simulink model "controlMCUSlugsMKII"  (Simulink 6.6)
settings: Solver=FixedStepDiscrete  StartTime=0.0  StopTime=10.0  FixedStep=0.01  RelTol=1e-3
InitFcn:
  | mcuInit
values from neighbouring files (symbols this model uses):
  apSampleTime = 0.01    [mcuInit.m]
  derivativesConstant = 5    [mcuInit.m]
  T = 0.01    [mcuInit.m]
undefined symbols (not defined in the file or in its folder): bankCommandLimit, baseHeight, bda, bde, bdr, bdt, bICda, bICde, bICdr, bICdt, controlMCUInit, daLimit, deLimit, drLimit, dtLimit, getAccBias, getAccels, getAttitude, getMidLevelCommands, getPassValues, getPidIdx, getVned, getWP, getXYZ, gsRead, ISA_g, lowRateTelemetryMavlink, mda, mde, mdr, mdt, mICda, mICde, mICdr, mICdt, pitchCommandLimit, protDecodeMavlink, readIpc, send2GS, setCurrentCommands, setDiagnosticFloat, setDiagnosticShort, setLogFloat1, setLogFloat2, setNavLat, setNavLong, setNavNav, u1, u2, updateEuler, updateLoad, updatePQR, updatePWM, updatePWM2, y1
libraries: dsPICdrivers x85, simulink x79, SLUGS_Library x23, aerolibconvert2 x5, aerolibutil x3
(part 5 of 5)

== system controlMCUSlugsMKII/Inner Loop/ Navigation/Navigation/Park, Deyst & How Lat Accel Cmd/GainSchedule L2 and Get Groundspeed/Norm  ==
  Vector : Inport
  Square Vx and Vy  Only. Vz is not considered CAREFUL : Subsystem  AncestorBlock=SLUGS_Library/Subsystem3
  Subsystem1 : SLUGS_Library/Subsystem1  SystemSampleTime=-1
  "[-25 25]" : Saturate  UpperLimit=25  LowerLimit=-25  SampleTime=.01
  Norm : Outport
  wires:
  Subsystem1/1 -> Norm/1
  Vector/1 -> "[-25 25]"/1
  Square Vx and Vy  Only. Vz is not considered CAREFUL/1(x dot y) -> Subsystem1/1
  "[-25 25]"/1 -> Square Vx and Vy  Only. Vz is not considered CAREFUL/1(x), Square Vx and Vy  Only. Vz is not considered CAREFUL/2(y)

== system controlMCUSlugsMKII/Inner Loop/ Navigation/Navigation/Park, Deyst & How Lat Accel Cmd/GainSchedule L2 and Get Groundspeed/Protect NaNs ==
  In1 : Inport
  Integer Delay3 : simulink/Discrete/Integer Delay  Orientation=left  vinit=0.0  samptime=T  NumDelays=1
  Relational Operator2 : RelationalOperator  Operator===  LogicOutDataTypeMode=Specify via dialog
  Switch3 : Switch  Criteria=u2 > Threshold  Threshold=0.3  SampleTime=.01
  Out1 : Outport  Orientation=down
  wires:
  Relational Operator2/1 -> Switch3/2
  In1/1 -> Switch3/1, Relational Operator2/1, Relational Operator2/2
  Switch3/1 -> Integer Delay3/1, Out1/1
  Integer Delay3/1 -> Switch3/3

== system controlMCUSlugsMKII/Inner Loop/ Navigation/Navigation/Park, Deyst & How Lat Accel Cmd/Park's Lateral Accel Command/Protect NaNs ==
  In1 : Inport
  Integer Delay3 : simulink/Discrete/Integer Delay  Orientation=left  vinit=0.0  samptime=T  NumDelays=1
  Relational Operator2 : RelationalOperator  Operator===  LogicOutDataTypeMode=Specify via dialog
  Switch3 : Switch  Criteria=u2 > Threshold  Threshold=0.3  SampleTime=.01
  Out1 : Outport  Orientation=down
  wires:
  Relational Operator2/1 -> Switch3/2
  In1/1 -> Switch3/1, Relational Operator2/1, Relational Operator2/2
  Switch3/1 -> Integer Delay3/1, Out1/1
  Integer Delay3/1 -> Switch3/3

== system controlMCUSlugsMKII/Inner Loop/ Navigation/Navigation/Compute WP Index/Compute P/Compute T  in Frenet/Normalize Vector ==
  Vector : Inport
  Divide : Product  Inputs=*/  OutScaling=2^-10
  Norm : Subsystem  AncestorBlock=SLUGS_Library/Navigation/Norm
  Zero Bound : Saturate  UpperLimit=inf  LowerLimit=0.001
  Normalized : Outport
  wires:
  Divide/1 -> Normalized/1
  Zero Bound/1 -> Divide/2
  Norm/1(Norm) -> Zero Bound/1
  Vector/1 -> Divide/1, Norm/1(Vector)

== system controlMCUSlugsMKII/Inner Loop/ Navigation/Navigation/Compute WP Index/Compute P/Geod2LTP1/ECEF2LTP (UEN) ==
  ECEF coordinates : Inport
  "Long, Lat" : Inport  Port=2
  Deg2R : Gain  Gain=pi/180  SaturateOnIntegerOverflow=on
  Demux3 : Demux  Outputs=2
  From Body to Universal1 : Subsystem
  Product1 : Product  Multiplication=Matrix(*)  SaturateOnIntegerOverflow=on  InputSameDT=on
  Out : Outport
  wires:
  "Long, Lat"/1 -> Deg2R/1
  Product1/1 -> Out/1
  Demux3/2 -> From Body to Universal1/2(lat)
  Demux3/1 -> From Body to Universal1/1(long)
  Deg2R/1 -> Demux3/1
  ECEF coordinates/1 -> Product1/2
  From Body to Universal1/1(DCM) -> Product1/1

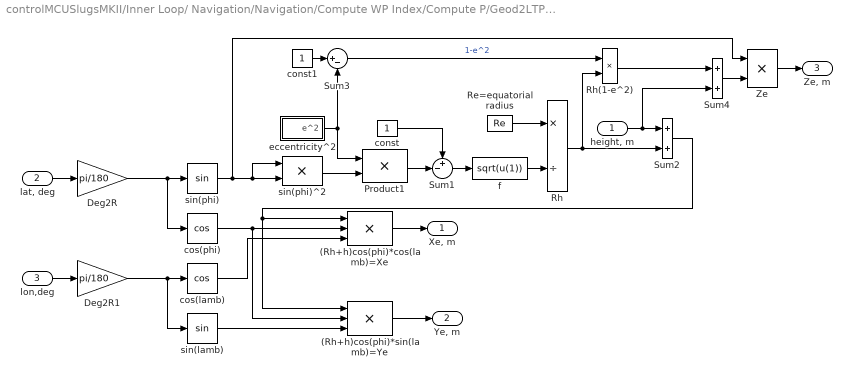
== system controlMCUSlugsMKII/Inner Loop/ Navigation/Navigation/Compute WP Index/Compute P/Geod2LTP1/Geod2ECEF1 ==
  "height, m" : Inport
  "lat, deg" : Inport  Port=2
  lon,deg : Inport  Port=3
  (Rh+h)cos(phi)*cos(lamb)=Xe : Product  Inputs=3  OutDataTypeMode=single  SaturateOnIntegerOverflow=on  InputSameDT=on
  (Rh+h)cos(phi)*sin(lamb)=Ye : Product  Inputs=3  OutDataTypeMode=single  SaturateOnIntegerOverflow=on  InputSameDT=on
  Deg2R : Gain  Gain=pi/180  OutDataTypeMode=Specify via dialog  OutDataType=float('single')  SaturateOnIntegerOverflow=on
  Deg2R1 : Gain  Gain=pi/180  OutDataTypeMode=Specify via dialog  OutDataType=float('single')  SaturateOnIntegerOverflow=on
  Product1 : Product  SaturateOnIntegerOverflow=on  InputSameDT=on
  Re=equatorial radius : Constant  Value=Re  OutDataTypeMode=single
  Rh : Product  Inputs=*/  OutDataTypeMode=single  SaturateOnIntegerOverflow=on  InputSameDT=on
  Rh(1-e^2) : Product  OutDataTypeMode=single  SaturateOnIntegerOverflow=on  InputSameDT=on
  Sum1 : Sum  Inputs=+-|  SaturateOnIntegerOverflow=on  InputSameDT=on
  Sum2 : Sum  SaturateOnIntegerOverflow=on  InputSameDT=on
      settings: AttributesFormatString=Rh+h
  Sum3 : Sum  Inputs=|+-  SaturateOnIntegerOverflow=on  InputSameDT=on
  Sum4 : Sum  OutDataTypeMode=single  SaturateOnIntegerOverflow=on  InputSameDT=on
      settings: AttributesFormatString=(1-e^2)Rh+h
  Ze : Product  OutDataTypeMode=single  SaturateOnIntegerOverflow=on  InputSameDT=on
  const : Constant  OutDataTypeMode=single
  const1 : Constant  OutDataTypeMode=single
  cos(lamb) : Trigonometry  Operator=cos
  cos(phi) : Trigonometry  Operator=cos
  eccentricity^2 : Subsystem
  f : Fcn  Expr=sqrt(u(1))
  sin(lamb) : Trigonometry
  sin(phi) : Trigonometry
  sin(phi)^2 : Product  SaturateOnIntegerOverflow=on  InputSameDT=on
  "Xe, m " : Outport
  "Ye, m " : Outport  Port=2
  "Ze, m " : Outport  Port=3
  wires:
  "lat, deg"/1 -> Deg2R/1
  sin(phi)/1 -> sin(phi)^2/1, sin(phi)^2/2, Ze/1
  f/1 -> Rh/2
  Re=equatorial radius/1 -> Rh/1
  Rh/1 -> Sum2/2, Rh(1-e^2)/2
  Product1/1 -> Sum1/2
  Sum1/1 -> f/1
  const/1 -> Sum1/1
  "height, m"/1 -> Sum4/2, Sum2/1
  eccentricity^2/1(e^2) -> Product1/1, Sum3/2
  sin(phi)^2/1 -> Product1/2
  const1/1 -> Sum3/1
  Sum3/1 -> Rh(1-e^2)/1  "1-e^2"
  Rh(1-e^2)/1 -> Sum4/1
  Sum4/1 -> Ze/2
  lon,deg/1 -> Deg2R1/1
  cos(phi)/1 -> (Rh+h)cos(phi)*cos(lamb)=Xe/2, (Rh+h)cos(phi)*sin(lamb)=Ye/2
  cos(lamb)/1 -> (Rh+h)cos(phi)*cos(lamb)=Xe/3
  sin(lamb)/1 -> (Rh+h)cos(phi)*sin(lamb)=Ye/3
  Ze/1 -> "Ze, m "/1
  Deg2R/1 -> cos(phi)/1, sin(phi)/1
  Deg2R1/1 -> cos(lamb)/1, sin(lamb)/1
  Sum2/1 -> (Rh+h)cos(phi)*sin(lamb)=Ye/1, (Rh+h)cos(phi)*cos(lamb)=Xe/1
  (Rh+h)cos(phi)*cos(lamb)=Xe/1 -> "Xe, m "/1
  (Rh+h)cos(phi)*sin(lamb)=Ye/1 -> "Ye, m "/1

== system controlMCUSlugsMKII/Inner Loop/ Navigation/Navigation/Compute WP Index/Compute P/Get Circles/Compute CCW Angle From 2 Vectors ==
  U : Inport
  V : Inport  Port=2
  Add : Sum  Inputs=+-  OutScaling=2^-10
  Embedded MATLAB Function1 : Stateflow chart
  Selector : Selector  IndexOptions=Index vector (dialog)  Indices=[1]  OutputSizes=1  InputPortWidth=3
  Selector1 : Selector  IndexOptions=Index vector (dialog)  Indices=[1]  OutputSizes=1  InputPortWidth=3
  Selector2 : Selector  IndexOptions=Index vector (dialog)  Indices=[2]  OutputSizes=1  InputPortWidth=3
  Selector3 : Selector  IndexOptions=Index vector (dialog)  Indices=[2]  OutputSizes=1  InputPortWidth=3
  Subsystem1 : SLUGS_Library/Subsystem4  SystemSampleTime=-1
  Subsystem4 : SLUGS_Library/Subsystem4  SystemSampleTime=-1
  CCW Ang : Outport
  wires:
  Embedded MATLAB Function1/1(angle) -> CCW Ang/1
  V/1 -> Selector1/1, Selector2/1
  U/1 -> Selector/1, Selector3/1
  Add/1 -> Embedded MATLAB Function1/1(rawAngle)
  Subsystem1/1 -> Add/2
  Subsystem4/1 -> Add/1
  Selector1/1 -> Subsystem1/2
  Selector2/1 -> Subsystem1/1
  Selector/1 -> Subsystem4/2
  Selector3/1 -> Subsystem4/1

== system controlMCUSlugsMKII/Inner Loop/ Navigation/Navigation/Compute WP Index/Compute P/Get Circles/Compute delta Left Turn ==
  gamma : Inport
  Enable : EnablePort
  Add : Sum  Inputs=+-  OutDataTypeMode=single  OutScaling=2^-10
  Constant1 : Constant  Value=2  OutDataTypeMode=single
  Constant5 : Constant  Value=pi  OutDataTypeMode=single
  Divide : Product  Inputs=*/  OutDataTypeMode=single  OutScaling=2^-10
  Gain : Gain  Gain=-1
  delta : Outport
  wires:
  Gain/1 -> delta/1
  Add/1 -> Divide/1
  gamma/1 -> Add/2
  Constant5/1 -> Add/1
  Divide/1 -> Gain/1
  Constant1/1 -> Divide/2

== system controlMCUSlugsMKII/Inner Loop/ Navigation/Navigation/Compute WP Index/Compute P/Get Circles/compute delta Right Turn ==
  gamma : Inport
  Enable : EnablePort
  Add : Sum  Inputs=-+  OutDataTypeMode=single  OutScaling=2^-10
  Constant1 : Constant  Value=2  OutDataTypeMode=single
  Constant5 : Constant  Value=pi  OutDataTypeMode=single
  Divide : Product  Inputs=*/  OutDataTypeMode=single  OutScaling=2^-10
  delta : Outport
  wires:
  Divide/1 -> delta/1  "delta"
  gamma/1 -> Add/2
  Constant1/1 -> Divide/2
  Add/1 -> Divide/1
  Constant5/1 -> Add/1

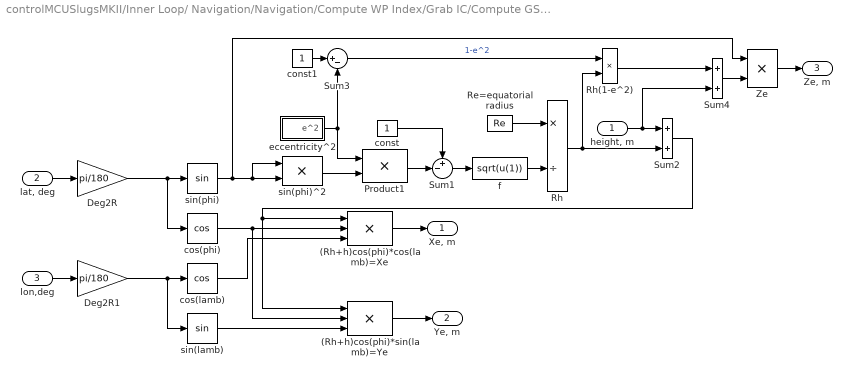
== system controlMCUSlugsMKII/Inner Loop/ Navigation/Navigation/Compute WP Index/Grab IC/Compute GS Location/Geod2ECEF1 ==
  "height, m" : Inport
  "lat, deg" : Inport  Port=2
  lon,deg : Inport  Port=3
  (Rh+h)cos(phi)*cos(lamb)=Xe : Product  Inputs=3  OutDataTypeMode=single  SaturateOnIntegerOverflow=on  InputSameDT=on
  (Rh+h)cos(phi)*sin(lamb)=Ye : Product  Inputs=3  OutDataTypeMode=single  SaturateOnIntegerOverflow=on  InputSameDT=on
  Deg2R : Gain  Gain=pi/180  OutDataTypeMode=Specify via dialog  OutDataType=float('single')  SaturateOnIntegerOverflow=on
  Deg2R1 : Gain  Gain=pi/180  OutDataTypeMode=Specify via dialog  OutDataType=float('single')  SaturateOnIntegerOverflow=on
  Product1 : Product  SaturateOnIntegerOverflow=on  InputSameDT=on
  Re=equatorial radius : Constant  Value=Re  OutDataTypeMode=single
  Rh : Product  Inputs=*/  OutDataTypeMode=single  SaturateOnIntegerOverflow=on  InputSameDT=on
  Rh(1-e^2) : Product  OutDataTypeMode=single  SaturateOnIntegerOverflow=on  InputSameDT=on
  Sum1 : Sum  Inputs=+-|  SaturateOnIntegerOverflow=on  InputSameDT=on
  Sum2 : Sum  SaturateOnIntegerOverflow=on  InputSameDT=on
      settings: AttributesFormatString=Rh+h
  Sum3 : Sum  Inputs=|+-  SaturateOnIntegerOverflow=on  InputSameDT=on
  Sum4 : Sum  OutDataTypeMode=single  SaturateOnIntegerOverflow=on  InputSameDT=on
      settings: AttributesFormatString=(1-e^2)Rh+h
  Ze : Product  OutDataTypeMode=single  SaturateOnIntegerOverflow=on  InputSameDT=on
  const : Constant  OutDataTypeMode=single
  const1 : Constant  OutDataTypeMode=single
  cos(lamb) : Trigonometry  Operator=cos
  cos(phi) : Trigonometry  Operator=cos
  eccentricity^2 : Subsystem
  f : Fcn  Expr=sqrt(u(1))
  sin(lamb) : Trigonometry
  sin(phi) : Trigonometry
  sin(phi)^2 : Product  SaturateOnIntegerOverflow=on  InputSameDT=on
  "Xe, m " : Outport
  "Ye, m " : Outport  Port=2
  "Ze, m " : Outport  Port=3
  wires:
  "lat, deg"/1 -> Deg2R/1
  sin(phi)/1 -> sin(phi)^2/1, sin(phi)^2/2, Ze/1
  f/1 -> Rh/2
  Re=equatorial radius/1 -> Rh/1
  Rh/1 -> Sum2/2, Rh(1-e^2)/2
  Product1/1 -> Sum1/2
  Sum1/1 -> f/1
  const/1 -> Sum1/1
  "height, m"/1 -> Sum4/2, Sum2/1
  eccentricity^2/1(e^2) -> Product1/1, Sum3/2
  sin(phi)^2/1 -> Product1/2
  const1/1 -> Sum3/1
  Sum3/1 -> Rh(1-e^2)/1  "1-e^2"
  Rh(1-e^2)/1 -> Sum4/1
  Sum4/1 -> Ze/2
  lon,deg/1 -> Deg2R1/1
  cos(phi)/1 -> (Rh+h)cos(phi)*cos(lamb)=Xe/2, (Rh+h)cos(phi)*sin(lamb)=Ye/2
  cos(lamb)/1 -> (Rh+h)cos(phi)*cos(lamb)=Xe/3
  sin(lamb)/1 -> (Rh+h)cos(phi)*sin(lamb)=Ye/3
  Ze/1 -> "Ze, m "/1
  Deg2R/1 -> cos(phi)/1, sin(phi)/1
  Deg2R1/1 -> cos(lamb)/1, sin(lamb)/1
  Sum2/1 -> (Rh+h)cos(phi)*sin(lamb)=Ye/1, (Rh+h)cos(phi)*cos(lamb)=Xe/1
  (Rh+h)cos(phi)*cos(lamb)=Xe/1 -> "Xe, m "/1
  (Rh+h)cos(phi)*sin(lamb)=Ye/1 -> "Ye, m "/1

== system controlMCUSlugsMKII/Inner Loop/ Navigation/Navigation/Compute WP Index/Switch when  in Line Segment/Compute  Projection/Protect NaNs ==
  In1 : Inport
  Integer Delay3 : simulink/Discrete/Integer Delay  Orientation=left  vinit=0.0  samptime=T  NumDelays=1
  Relational Operator2 : RelationalOperator  Operator===  LogicOutDataTypeMode=Specify via dialog
  Switch3 : Switch  Criteria=u2 > Threshold  Threshold=0.3  SampleTime=.01
  Out1 : Outport  Orientation=down
  wires:
  Relational Operator2/1 -> Switch3/2
  In1/1 -> Switch3/1, Relational Operator2/1, Relational Operator2/2
  Switch3/1 -> Integer Delay3/1, Out1/1
  Integer Delay3/1 -> Switch3/3

== system controlMCUSlugsMKII/Inner Loop/ Navigation/Navigation/Compute WP Index/Switch when  in Line Segment/Compute  Projection/Subsystem3 ==
  x : Inport
  y : Inport  Port=2
  Embedded MATLAB Function : Stateflow chart
  x dot y : Outport
  wires:
  Embedded MATLAB Function/1(xDoty) -> x dot y/1
  x/1 -> Embedded MATLAB Function/1(x)
  y/1 -> Embedded MATLAB Function/2(y)

== system controlMCUSlugsMKII/Inner Loop/ Navigation/Navigation/Compute WP Index/Switch when  in Line Segment/Compute Total Run/Compute Distance ==
  Pos 1 : Inport
  Pos 2 : Inport  Port=2
  Add : Sum  Inputs=+-  OutScaling=2^-10
  Norm : Subsystem  AncestorBlock=SLUGS_Library/Navigation/Norm
  Dist : Outport
  wires:
  Norm/1(Norm) -> Dist/1
  Add/1 -> Norm/1(Vector)
  Pos 2/1 -> Add/2
  Pos 1/1 -> Add/1

== system controlMCUSlugsMKII/Inner Loop/ Navigation/Navigation/Compute WP Index/Switch when  in Line Segment/Compute Total Run/Protect NaNs ==
  In1 : Inport
  Integer Delay3 : simulink/Discrete/Integer Delay  Orientation=left  vinit=0.0  samptime=T  NumDelays=1
  Relational Operator2 : RelationalOperator  Operator===  LogicOutDataTypeMode=Specify via dialog
  Switch3 : Switch  Criteria=u2 > Threshold  Threshold=0.3  SampleTime=.01
  Out1 : Outport  Orientation=down
  wires:
  Relational Operator2/1 -> Switch3/2
  In1/1 -> Switch3/1, Relational Operator2/1, Relational Operator2/2
  Switch3/1 -> Integer Delay3/1, Out1/1
  Integer Delay3/1 -> Switch3/3

== system controlMCUSlugsMKII/Inner Loop/ Navigation/Navigation/Compute WP Index/Switch when  in Line Segment/WP Update/Detect Change ==
  Data : Inport
  Difference1 : simulink/Discrete/Difference  SystemSampleTime=-1  ICPrevInput=0.0  OutDataType=sfix(16)  OutScaling=2^-10  DoSatur=off
  Saturation1 : Saturate  UpperLimit=1  LowerLimit=0  SampleTime=T
  Subsystem9 : SLUGS_Library/Subsystem9  SystemSampleTime=-1
  change? : Outport
  wires:
  Subsystem9/1 -> Saturation1/1
  Saturation1/1 -> change?/1
  Data/1 -> Difference1/1
  Difference1/1 -> Subsystem9/1

== system controlMCUSlugsMKII/Inner Loop/ Navigation/Navigation/Compute WP Index/Switch when  in Line Segment/WP Update/Detect Change1 ==
  Data : Inport
  Difference1 : simulink/Discrete/Difference  SystemSampleTime=-1  ICPrevInput=0.0  OutDataType=sfix(16)  OutScaling=2^-10  DoSatur=off
  Saturation1 : Saturate  UpperLimit=1  LowerLimit=0  SampleTime=T
  Subsystem9 : SLUGS_Library/Subsystem9  SystemSampleTime=-1
  change? : Outport
  wires:
  Difference1/1 -> Subsystem9/1
  Data/1 -> Difference1/1
  Saturation1/1 -> change?/1
  Subsystem9/1 -> Saturation1/1

== system controlMCUSlugsMKII/Inner Loop/ Navigation/Navigation/Compute WP Index/Switch when  in Line Segment/WP Update/Detect Change2 ==
  Data : Inport
  Difference1 : simulink/Discrete/Difference  SystemSampleTime=-1  ICPrevInput=0.0  OutDataType=sfix(16)  OutScaling=2^-10  DoSatur=off
  Saturation1 : Saturate  UpperLimit=1  LowerLimit=0  SampleTime=T
  Subsystem9 : SLUGS_Library/Subsystem9  SystemSampleTime=-1
  change? : Outport
  wires:
  Subsystem9/1 -> Saturation1/1
  Saturation1/1 -> change?/1
  Data/1 -> Difference1/1
  Difference1/1 -> Subsystem9/1

== system controlMCUSlugsMKII/Inner Loop/ Navigation/Navigation/Get Wps Compute Frenet/Geod2LTP1/ECEF2LTP (UEN)/From Body to Universal1 ==
  long : Inport
  lat : Inport  Port=2
  Mux : Mux  Inputs=2
  Reshape 9x1->3x1 : S-Function  FunctionName=sreshape  Parameters=OutputDimensionality, OutputDimensions  mask(Reshape){OutputDimensionality=Customize, OutputDimensions=[3,3]}
      mask prompts: OutputDimensionality "Output dimensionality:"; OutputDimensions "Output dimensions:"
      mask help:
      | Change the dimensions of a vector or matrix input signal. Output
      |  - a one-dimensional array (vector),
      |  - a column vector (Mx1 matrix),
      |  - a row vector (1xN matrix), or
      |  - a matrix or vector with specified dimensions, e.g., [M, N] or [W].
      mask init:
      | s = reshapemask(gcb,'init');
      mask StyleString: popup(1-D array|Column vector|Row vector|Customize),edit
      mask CallbackString: reshapemask(gcb,'cbDimensionality')|
      mask Display: disp('Reshape')
  Rotation Matrix from Long//Lat : Subsystem
      mask Type: Vector Transformation
      mask Description: Vector Transformation
      mask Display: disp('axis')
  DCM : Outport
  wires:
  lat/1 -> Mux/2
  long/1 -> Mux/1
  Mux/1 -> Rotation Matrix from Long//Lat/1(long lat)
  Rotation Matrix from Long//Lat/1(DCM) -> Reshape 9x1->3x1/1
  Reshape 9x1->3x1/1 -> DCM/1

== system controlMCUSlugsMKII/Inner Loop/ Navigation/Navigation/Get Wps Compute Frenet/Geod2LTP1/Geod2ECEF1/eccentricity^2 ==
  " " : Product  OutDataTypeMode=single  SaturateOnIntegerOverflow=on  InputSameDT=on
  Re=equatorial radius1 : Constant  Value=Re  OutDataTypeMode=single
  Rp=polar radius : Constant  Value=Rp  OutDataTypeMode=single
  Sum5 : Sum  Inputs=|+-  SaturateOnIntegerOverflow=on  InputSameDT=on
  const2 : Constant  OutDataTypeMode=single
  e^1 : Product  Inputs=*/  OutDataTypeMode=single  SaturateOnIntegerOverflow=on  InputSameDT=on
  e^2 : Outport
  wires:
  Re=equatorial radius1/1 -> e^1/2
  Rp=polar radius/1 -> e^1/1
  const2/1 -> Sum5/1
  e^1/1 -> " "/2, " "/1
  " "/1 -> Sum5/2
  Sum5/1 -> e^2/1

== system controlMCUSlugsMKII/Inner Loop/ Navigation/Navigation/Get Wps Compute Frenet/Geod2LTP2/ECEF2LTP (UEN)/From Body to Universal1 ==
  long : Inport
  lat : Inport  Port=2
  Mux : Mux  Inputs=2
  Reshape 9x1->3x1 : S-Function  FunctionName=sreshape  Parameters=OutputDimensionality, OutputDimensions  mask(Reshape){OutputDimensionality=Customize, OutputDimensions=[3,3]}
      mask prompts: OutputDimensionality "Output dimensionality:"; OutputDimensions "Output dimensions:"
      mask help:
      | Change the dimensions of a vector or matrix input signal. Output
      |  - a one-dimensional array (vector),
      |  - a column vector (Mx1 matrix),
      |  - a row vector (1xN matrix), or
      |  - a matrix or vector with specified dimensions, e.g., [M, N] or [W].
      mask init:
      | s = reshapemask(gcb,'init');
      mask StyleString: popup(1-D array|Column vector|Row vector|Customize),edit
      mask CallbackString: reshapemask(gcb,'cbDimensionality')|
      mask Display: disp('Reshape')
  Rotation Matrix from Long//Lat : Subsystem
      mask Type: Vector Transformation
      mask Description: Vector Transformation
      mask Display: disp('axis')
  DCM : Outport
  wires:
  lat/1 -> Mux/2
  long/1 -> Mux/1
  Mux/1 -> Rotation Matrix from Long//Lat/1(long lat)
  Rotation Matrix from Long//Lat/1(DCM) -> Reshape 9x1->3x1/1
  Reshape 9x1->3x1/1 -> DCM/1

== system controlMCUSlugsMKII/Inner Loop/ Navigation/Navigation/Get Wps Compute Frenet/Geod2LTP2/Geod2ECEF1/eccentricity^2 ==
  " " : Product  OutDataTypeMode=single  SaturateOnIntegerOverflow=on  InputSameDT=on
  Re=equatorial radius1 : Constant  Value=Re  OutDataTypeMode=single
  Rp=polar radius : Constant  Value=Rp  OutDataTypeMode=single
  Sum5 : Sum  Inputs=|+-  SaturateOnIntegerOverflow=on  InputSameDT=on
  const2 : Constant  OutDataTypeMode=single
  e^1 : Product  Inputs=*/  OutDataTypeMode=single  SaturateOnIntegerOverflow=on  InputSameDT=on
  e^2 : Outport
  wires:
  Re=equatorial radius1/1 -> e^1/2
  Rp=polar radius/1 -> e^1/1
  const2/1 -> Sum5/1
  e^1/1 -> " "/2, " "/1
  " "/1 -> Sum5/2
  Sum5/1 -> e^2/1

== system controlMCUSlugsMKII/Inner Loop/ Navigation/Navigation/Park, Deyst & How Lat Accel Cmd/Compute Eta/Subsystem6/Protect NaNs ==
  In1 : Inport
  Integer Delay3 : simulink/Discrete/Integer Delay  Orientation=left  vinit=0.0  samptime=T  NumDelays=1
  Relational Operator2 : RelationalOperator  Operator===  LogicOutDataTypeMode=Specify via dialog
  Switch3 : Switch  Criteria=u2 > Threshold  Threshold=0.3  SampleTime=.01
  Out1 : Outport  Orientation=down
  wires:
  Relational Operator2/1 -> Switch3/2
  In1/1 -> Switch3/1, Relational Operator2/1, Relational Operator2/2
  Switch3/1 -> Integer Delay3/1, Out1/1
  Integer Delay3/1 -> Switch3/3

== system controlMCUSlugsMKII/Inner Loop/ Navigation/Navigation/Park, Deyst & How Lat Accel Cmd/GainSchedule L2 and Get Groundspeed/Norm /Square Vx and Vy  Only. Vz is not considered CAREFUL ==
  x : Inport
  y : Inport  Port=2
  Embedded MATLAB Function : Stateflow chart
  x dot y : Outport
  wires:
  x/1 -> Embedded MATLAB Function/1(x)
  y/1 -> Embedded MATLAB Function/2(y)
  Embedded MATLAB Function/1(xDoty) -> x dot y/1

== system controlMCUSlugsMKII/Inner Loop/ Navigation/Navigation/Compute WP Index/Compute P/Compute T  in Frenet/Normalize Vector/Norm ==
  Vector : Inport
  Subsystem1 : SLUGS_Library/Subsystem1  SystemSampleTime=-1
  Subsystem3 : Subsystem  AncestorBlock=SLUGS_Library/Subsystem3
  Norm : Outport
  wires:
  Subsystem3/1(x dot y) -> Subsystem1/1
  Vector/1 -> Subsystem3/2(y), Subsystem3/1(x)
  Subsystem1/1 -> Norm/1

== system controlMCUSlugsMKII/Inner Loop/ Navigation/Navigation/Compute WP Index/Compute P/Geod2LTP1/ECEF2LTP (UEN)/From Body to Universal1 ==
  long : Inport
  lat : Inport  Port=2
  Mux : Mux  Inputs=2
  Reshape 9x1->3x1 : S-Function  FunctionName=sreshape  Parameters=OutputDimensionality, OutputDimensions  mask(Reshape){OutputDimensionality=Customize, OutputDimensions=[3,3]}
      mask prompts: OutputDimensionality "Output dimensionality:"; OutputDimensions "Output dimensions:"
      mask help:
      | Change the dimensions of a vector or matrix input signal. Output
      |  - a one-dimensional array (vector),
      |  - a column vector (Mx1 matrix),
      |  - a row vector (1xN matrix), or
      |  - a matrix or vector with specified dimensions, e.g., [M, N] or [W].
      mask init:
      | s = reshapemask(gcb,'init');
      mask StyleString: popup(1-D array|Column vector|Row vector|Customize),edit
      mask CallbackString: reshapemask(gcb,'cbDimensionality')|
      mask Display: disp('Reshape')
  Rotation Matrix from Long//Lat : Subsystem
      mask Type: Vector Transformation
      mask Description: Vector Transformation
      mask Display: disp('axis')
  DCM : Outport
  wires:
  lat/1 -> Mux/2
  long/1 -> Mux/1
  Mux/1 -> Rotation Matrix from Long//Lat/1(long lat)
  Rotation Matrix from Long//Lat/1(DCM) -> Reshape 9x1->3x1/1
  Reshape 9x1->3x1/1 -> DCM/1

== system controlMCUSlugsMKII/Inner Loop/ Navigation/Navigation/Compute WP Index/Compute P/Geod2LTP1/Geod2ECEF1/eccentricity^2 ==
  " " : Product  OutDataTypeMode=single  SaturateOnIntegerOverflow=on  InputSameDT=on
  Re=equatorial radius1 : Constant  Value=Re  OutDataTypeMode=single
  Rp=polar radius : Constant  Value=Rp  OutDataTypeMode=single
  Sum5 : Sum  Inputs=|+-  SaturateOnIntegerOverflow=on  InputSameDT=on
  const2 : Constant  OutDataTypeMode=single
  e^1 : Product  Inputs=*/  OutDataTypeMode=single  SaturateOnIntegerOverflow=on  InputSameDT=on
  e^2 : Outport
  wires:
  Re=equatorial radius1/1 -> e^1/2
  Rp=polar radius/1 -> e^1/1
  const2/1 -> Sum5/1
  e^1/1 -> " "/2, " "/1
  " "/1 -> Sum5/2
  Sum5/1 -> e^2/1

== system controlMCUSlugsMKII/Inner Loop/ Navigation/Navigation/Compute WP Index/Grab IC/Compute GS Location/Geod2ECEF1/eccentricity^2 ==
  " " : Product  OutDataTypeMode=single  SaturateOnIntegerOverflow=on  InputSameDT=on
  Re=equatorial radius1 : Constant  Value=Re  OutDataTypeMode=single
  Rp=polar radius : Constant  Value=Rp  OutDataTypeMode=single
  Sum5 : Sum  Inputs=|+-  SaturateOnIntegerOverflow=on  InputSameDT=on
  const2 : Constant  OutDataTypeMode=single
  e^1 : Product  Inputs=*/  OutDataTypeMode=single  SaturateOnIntegerOverflow=on  InputSameDT=on
  e^2 : Outport
  wires:
  Re=equatorial radius1/1 -> e^1/2
  Rp=polar radius/1 -> e^1/1
  const2/1 -> Sum5/1
  e^1/1 -> " "/2, " "/1
  " "/1 -> Sum5/2
  Sum5/1 -> e^2/1

== system controlMCUSlugsMKII/Inner Loop/ Navigation/Navigation/Compute WP Index/Switch when  in Line Segment/Compute Total Run/Compute Distance/Norm ==
  Vector : Inport
  Subsystem1 : SLUGS_Library/Subsystem1  SystemSampleTime=-1
  Subsystem3 : Subsystem  AncestorBlock=SLUGS_Library/Subsystem3
  Norm : Outport
  wires:
  Subsystem1/1 -> Norm/1
  Vector/1 -> Subsystem3/1(x), Subsystem3/2(y)
  Subsystem3/1(x dot y) -> Subsystem1/1

== system controlMCUSlugsMKII/Inner Loop/ Navigation/Navigation/Get Wps Compute Frenet/Geod2LTP1/ECEF2LTP (UEN)/From Body to Universal1/Rotation Matrix from Long//Lat ==
  note: Calculate Coefficients of DCM Row-Wise
  long lat : Inport
  11 : Fcn  Expr=cos(u[1])*cos(u[2])
  12 : Fcn  Expr=sin(u[1])*cos(u[2])
  13 : Fcn  Expr=sin(u[2])
  21 : Fcn  Expr=-sin(u[1])
  22 : Fcn  Expr=cos(u[1])
  23 : Fcn  Expr=0
  31 : Fcn  Expr=-sin(u[2])*cos(u[1])
  32 : Fcn  Expr=-sin(u[1])*sin(u[2])
  33 : Fcn  Expr=cos(u[2])
  Mux2 : Mux  Inputs=9
  DCM : Outport  InitialOutput=0
  wires:
  33/1 -> Mux2/9
  23/1 -> Mux2/8
  13/1 -> Mux2/7
  32/1 -> Mux2/6
  22/1 -> Mux2/5
  12/1 -> Mux2/4
  31/1 -> Mux2/3
  21/1 -> Mux2/2
  11/1 -> Mux2/1
  Mux2/1 -> DCM/1
  long lat/1 -> 11/1, 33/1, 23/1, 13/1, 32/1, 22/1, 12/1, 31/1, 21/1

== system controlMCUSlugsMKII/Inner Loop/ Navigation/Navigation/Get Wps Compute Frenet/Geod2LTP2/ECEF2LTP (UEN)/From Body to Universal1/Rotation Matrix from Long//Lat ==
  note: Calculate Coefficients of DCM Row-Wise
  long lat : Inport
  11 : Fcn  Expr=cos(u[1])*cos(u[2])
  12 : Fcn  Expr=sin(u[1])*cos(u[2])
  13 : Fcn  Expr=sin(u[2])
  21 : Fcn  Expr=-sin(u[1])
  22 : Fcn  Expr=cos(u[1])
  23 : Fcn  Expr=0
  31 : Fcn  Expr=-sin(u[2])*cos(u[1])
  32 : Fcn  Expr=-sin(u[1])*sin(u[2])
  33 : Fcn  Expr=cos(u[2])
  Mux2 : Mux  Inputs=9
  DCM : Outport  InitialOutput=0
  wires:
  33/1 -> Mux2/9
  23/1 -> Mux2/8
  13/1 -> Mux2/7
  32/1 -> Mux2/6
  22/1 -> Mux2/5
  12/1 -> Mux2/4
  31/1 -> Mux2/3
  21/1 -> Mux2/2
  11/1 -> Mux2/1
  Mux2/1 -> DCM/1
  long lat/1 -> 11/1, 33/1, 23/1, 13/1, 32/1, 22/1, 12/1, 31/1, 21/1

== system controlMCUSlugsMKII/Inner Loop/ Navigation/Navigation/Compute WP Index/Compute P/Compute T  in Frenet/Normalize Vector/Norm/Subsystem3 ==
  x : Inport
  y : Inport  Port=2
  Dot Product : simulink/Math Operations/Dot Product  InputSameDT=on  OutDataType=sfix(16)  OutScaling=2^-10  DoSatur=off
  Embedded MATLAB Function : Stateflow chart
  Environment Controller : simulink/Signal Routing/Environment Controller  SystemSampleTime=-1
  x dot y : Outport
  wires:
  y/1 -> Embedded MATLAB Function/2(y), Dot Product/2
  x/1 -> Embedded MATLAB Function/1(x), Dot Product/1
  Dot Product/1 -> Environment Controller/1
  Embedded MATLAB Function/1(xDoty) -> Environment Controller/2
  Environment Controller/1 -> x dot y/1

== system controlMCUSlugsMKII/Inner Loop/ Navigation/Navigation/Compute WP Index/Compute P/Geod2LTP1/ECEF2LTP (UEN)/From Body to Universal1/Rotation Matrix from Long//Lat ==
  note: Calculate Coefficients of DCM Row-Wise
  long lat : Inport
  11 : Fcn  Expr=cos(u[1])*cos(u[2])
  12 : Fcn  Expr=sin(u[1])*cos(u[2])
  13 : Fcn  Expr=sin(u[2])
  21 : Fcn  Expr=-sin(u[1])
  22 : Fcn  Expr=cos(u[1])
  23 : Fcn  Expr=0
  31 : Fcn  Expr=-sin(u[2])*cos(u[1])
  32 : Fcn  Expr=-sin(u[1])*sin(u[2])
  33 : Fcn  Expr=cos(u[2])
  Mux2 : Mux  Inputs=9
  DCM : Outport  InitialOutput=0
  wires:
  33/1 -> Mux2/9
  23/1 -> Mux2/8
  13/1 -> Mux2/7
  32/1 -> Mux2/6
  22/1 -> Mux2/5
  12/1 -> Mux2/4
  31/1 -> Mux2/3
  21/1 -> Mux2/2
  11/1 -> Mux2/1
  Mux2/1 -> DCM/1
  long lat/1 -> 11/1, 33/1, 23/1, 13/1, 32/1, 22/1, 12/1, 31/1, 21/1

== system controlMCUSlugsMKII/Inner Loop/ Navigation/Navigation/Compute WP Index/Switch when  in Line Segment/Compute Total Run/Compute Distance/Norm/Subsystem3 ==
  x : Inport
  y : Inport  Port=2
  Embedded MATLAB Function : Stateflow chart
  x dot y : Outport
  wires:
  x/1 -> Embedded MATLAB Function/1(x)
  y/1 -> Embedded MATLAB Function/2(y)
  Embedded MATLAB Function/1(xDoty) -> x dot y/1

== matlab function myMux Fun1 ==
  data: u1 input inherited; y output inherited; u2 input inherited; u3 input inherited; u4 input inherited
function y = myMux(u1, u2, u3, u4 )
% This block supports an embeddable subset of the MATLAB language.
% See the help menu for details. 

y = [u1(1); u2(1); u3(1); u4(1)];

== matlab function Update PWM Commands and Send Telemetry/Generate PWM Signals Based on the Control Type/If  Control Type Is Manual/myMux Fun1 ==
  data: u1 input inherited; y output inherited; u2 input inherited; u3 input inherited; u4 input inherited
function y = myMux(u1, u2, u3, u4 )
% This block supports an embeddable subset of the MATLAB language.
% See the help menu for details. 

y = [u1(1); u2(1); u3(1); u4(1)];

== matlab function Trim Vals/Control Surface Input/myMux Fun5 ==
  data: u1 input inherited; y output inherited; u2 input inherited; u3 input inherited; u4 input inherited; u5 input inherited
function y = myMux(u1, u2, u3, u4, u5)
% This block supports an embeddable subset of the MATLAB language.
% See the help menu for details. 

y = [u1(1); u2(1); u3(1); u4(1); u5(1)];

== matlab function Trim Vals/Bufffer IC/Buffer IC Channel ==
  data: latest input inherited; history output inherited
function history = bufferICValues(latest)
% This block supports an embeddable subset of the MATLAB language.
% See the help menu for details. 

persistent oldValues;

if isempty(oldValues)
    oldValues = uint16([0 0 0 0 0 0 0]);
end

history = uint16([0 0 0 0 0 0 0]);

for i=7:-1:2
    oldValues(i) = oldValues(i-1);
	history(i) = oldValues(i-1);
end
	
oldValues(1) = latest;
history(1) = latest;

== matlab function Inner Loop/ Navigation/Navigation/Compute WP Index/Compute P/Compute T in Frenet/Normalize Vector/Norm/Subsystem3/Embedded MATLAB Function ==
  data: x input inherited; y input inherited; xDoty output inherited
function xDoty = myDot(x,y)
% This block supports an embeddable subset of the MATLAB language.
% See the help menu for details. 

xDoty = x(1)*y(1) + x(2)*y(2) + x(3)*y(3);

== matlab function Trim Vals/Bufffer IC/Buffer IC Channel1 ==
  data: latest input inherited; history output inherited
function history = bufferICValues(latest)
% This block supports an embeddable subset of the MATLAB language.
% See the help menu for details. 

persistent oldValues;

if isempty(oldValues)
    oldValues = uint16([0 0 0 0 0 0 0]);
end

history = uint16([0 0 0 0 0 0 0]);

for i=7:-1:2
    oldValues(i) = oldValues(i-1);
	history(i) = oldValues(i-1);
end
	
oldValues(1) = latest;
history(1) = latest;

== matlab function Inner Loop/ Navigation/Longitudinal Channel/Compute Airspeed/Subsystem1/negprotect ==
  data: val input inherited; zpVal output inherited
function zpVal = negProt(val)
% This block supports an embeddable subset of the MATLAB language.
% See the help menu for details. 

if val >= single(0.001)
    zpVal = val;
else
    zpVal = single(0.001);
end

== matlab function Inner Loop/ Navigation/Navigation/Compute WP Index/Compute P/Get Circles/Compute Circles ==
  data: sd input inherited; O output inherited; cd input inherited; WP1 input inherited; R input inherited; T1 input inherited; P output inherited; Pch output inherited; T2 input inherited; PchB output inherited
function [O,P,Pch, PchB] = getO(sd, cd, WP1, R, T1, T2)
    % This block supports an embeddable subset of the MATLAB language.
    % See the help menu for details.

    % rotate the vector delta degrees
    r_vec = zeros(3,1);
    r_vec(1) = -T1(1)*cd -T1(2)*sd;
    r_vec(2) = T1(1)*sd -T1(2)*cd;

    %compute M
    if localAbs(sd)>0.01
        M = localAbs(R/sd);
    else
        M = single(0);
    end

    %find the distance from WP
    P = M*cd;

    % find the center of the circle
    O = WP1 + r_vec.*M;

    % find the tangent points
    Pch = WP1-T1*P;
    PchB = WP1 + T2*P;
end

function absVal = localAbs(x)
    if x < 0
        absVal = single(-1*x);
    else
        absVal = single(x);
    end
end

== matlab function Inner Loop/ Navigation/Navigation/Compute WP Index/Compute P/Get Circles/Compute CCW Angle From 2 Vectors/Embedded MATLAB Function1 ==
  data: rawAngle input inherited; angle output inherited
function angle = mapToTwoPi(rawAngle)

 if(rawAngle < 0)
  angle = rawAngle + 2*pi;
 else
  angle = rawAngle;   
 end

== matlab function Inner Loop/ Navigation/Navigation/Compute WP Index/Embedded MATLAB Function ==
  data: wpStart input inherited; wpCount input inherited; wp0 output inherited; swIncrement input inherited; wp1 output inherited; wp2 output inherited; wpEnabl input inherited
function [wp0,wp1, wp2] = getNextWP(wpStart, wpCount, swIncrement, wpEnabl)

% Declare static variables
persistent fromWP;
persistent toWP;
persistent totoWP;

%initialize the static variables
if isempty(fromWP)
    fromWP = uint8(wpStart);
    toWP = uint8(fromWP+1);
    % check if there are more than 2 WPs
    if wpCount > toWP + 1
        totoWP = uint8(toWP+1);
    else
        totoWP = uint8(fromWP);
    end
end

%if WP Nav was just enabled
if wpEnabl == 1
    fromWP = uint8(0);
    toWP = uint8(1);
    totoWP = uint8(2);
end;

% if there is a change of wp
if swIncrement == 1
    fromWP = toWP;
    toWP = totoWP;
    totoWP = totoWP +1;
    if (totoWP>wpCount)
        totoWP = wpStart;
    end
end

wp0 = fromWP;
wp1 = toWP;
wp2 = totoWP;

== matlab function Inner Loop/ Navigation/Navigation/Compute WP Index/Embedded MATLAB Function1 ==
  data: swDistanceRdy input inherited; timeLimit input inherited; swIncrement output inherited
function swIncrement  = computeSwitch(swDistanceRdy, timeLimit)

% Declare static variables
persistent oldSw;
persistent internalTimer;

%initialize the static variables
if isempty(oldSw)
    oldSw = uint8(0);
    internalTimer = uint16(0);
    % check if there are more than 2 WPs
end 

swIncrement = 0;

%if we just had a flip
if swDistanceRdy == 1 && oldSw == 0
    % if enough time has passed that another switch is valid
    if internalTimer > timeLimit
        swIncrement = 1;
        internalTimer = uint16(0);
    end
end;

internalTimer = internalTimer +1;
oldSw = swDistanceRdy;

== matlab function Inner Loop/ Navigation/Longitudinal Channel/myMux Fun1 ==
  data: u1 input inherited; y output inherited; u2 input inherited
function y = myMux(u1, u2)
% This block supports an embeddable subset of the MATLAB language.
% See the help menu for details. 

y = [u1(1); u2(1)];

== matlab function Inner Loop/ Navigation/myMux Fun2 ==
  data: u1 input inherited; y output inherited; u2 input inherited; u3 input inherited
function y = myMux(u1, u2, u3)
% This block supports an embeddable subset of the MATLAB language.
% See the help menu for details. 

y = [u1(1); u2(1); u3(1)];

== matlab function Inner Loop/ Navigation/Longitudinal Channel/0.5 sec  tau for Turns/Embedded MATLAB Function ==
  data: u input inherited; y output inherited; T input inherited; f input inherited
function y = fcn(u,T,f)
% This block supports an embeddable subset of the MATLAB language.
% See the help menu for details. 

persistent a
persistent b
persistent y_km1
persistent u_km1
if isempty(a)
    %tf = [T*omega/(2+T*omega) T*omega/(2+T*omega)],[1 (T*omega-2)/(T*omega+2)]
    %tf = [a a],[1 -b]
    omega = 2*pi*f;
    a=T*omega/(2+T*omega);
    b=-(T*omega-2)/(T*omega+2);
    y_km1=u;
    u_km1=u;
end

y = a*(u+u_km1)+b*y_km1;
y_km1=y;
u_km1=u;

== matlab function Inner Loop/ Navigation/Lateral Channel/Sideslip Compensation/Bank to Psi Dot/negprotect ==
  data: val input inherited; zpVal output inherited
function zpVal = negProt(val)
% This block supports an embeddable subset of the MATLAB language.
% See the help menu for details. 

if val >= single(0.001)
    zpVal = val;
else
    zpVal = single(0.001);
end

== matlab function Inner Loop/ Navigation/Navigation/Park, Deyst & How Lat Accel Cmd/Compute Eta/negprotect ==
  data: val input inherited; zpVal output inherited
function zpVal = negProt(val)
% This block supports an embeddable subset of the MATLAB language.
% See the help menu for details. 

if val >= single(0.001)
    zpVal = val;
else
    zpVal = single(0.001);
end

== matlab function Inner Loop/ Navigation/Navigation/Park, Deyst & How Lat Accel Cmd/GainSchedule L2 and Get Groundspeed/Norm /Square Vx and Vy Only. Vz is not considered CAREFUL/Embedded MATLAB Function ==
  data: x input inherited; y input inherited; xDoty output inherited
function xDoty = myDot(x,y)
% This block supports an embeddable subset of the MATLAB language.
% See the help menu for details. 

xDoty = x(1)*y(1) + x(2)*y(2);

== matlab function Inner Loop/ Navigation/Lateral Channel/myMux Fun1 ==
  data: u1 input inherited; y output inherited; u2 input inherited; u3 input inherited
function y = myMux(u1, u2, u3)
% This block supports an embeddable subset of the MATLAB language.
% See the help menu for details. 

y = [u1(1); u2(1); u3(1)];

== matlab function Inner Loop/ Navigation/Navigation/Compute WP Index/myMux Fun2 ==
  data: u1 input inherited; y output inherited; u2 input inherited; u3 input inherited; u4 input inherited
function y = myMux(u1, u2, u3, u4)
% This block supports an embeddable subset of the MATLAB language.
% See the help menu for details. 

y = [u1(1); u2(1); u3(1); u4(1)];

== matlab function Update PWM Commands and Send Telemetry/Generate PWM Signals Based on the Control Type/If  Control Type Is Wp Follow or Inner Cmds/myMux Fun1 ==
  data: u1 input inherited; y output inherited; u2 input inherited; u3 input inherited; u4 input inherited
function y = myMux(u1, u2, u3, u4 )
% This block supports an embeddable subset of the MATLAB language.
% See the help menu for details. 

y = [u1(1); u2(1); u3(1); u4(1)];

== matlab function Update PWM Commands and Send Telemetry/Generate PWM Signals Based on the Control Type/If  Control Type Is Passthrough/myMux Fun1 ==
  data: u1 input inherited; y output inherited; u2 input inherited; u3 input inherited; u4 input inherited
function y = myMux(u1, u2, u3, u4 )
% This block supports an embeddable subset of the MATLAB language.
% See the help menu for details. 

y = [u1(1); u2(1); u3(1); u4(1)];

== matlab function Update PWM Commands and Send Telemetry/Generate PWM Signals Based on the Control Type/If  Control Type Is Selective Passthrough/myMux Fun1 ==
  data: u1 input inherited; y output inherited; u2 input inherited; u3 input inherited; u4 input inherited
function y = myMux(u1, u2, u3, u4 )
% This block supports an embeddable subset of the MATLAB language.
% See the help menu for details. 

y = [u1(1); u2(1); u3(1); u4(1)];

== matlab function Update PWM Commands and Send Telemetry/myMux Fun1 ==
  data: u1 input inherited; y output inherited; u2 input inherited
function y = myMux(u1, u2)
% This block supports an embeddable subset of the MATLAB language.
% See the help menu for details. 

y = [u1(1:4); u2(1)];

== matlab function get Nav Vars/Embedded MATLAB Function ==
  data: u input inherited; y output inherited
function y = TwoPi(u)
% This block supports an embeddable subset of the MATLAB language.
% See the help menu for details. 

if ( u < 0 )
    y = u + 2*pi;
else
    y = u;
end

== matlab function Trim Vals/Bufffer IC/Buffer IC Channel2 ==
  data: latest input inherited; history output inherited
function history = bufferICValues(latest)
% This block supports an embeddable subset of the MATLAB language.
% See the help menu for details. 

persistent oldValues;

if isempty(oldValues)
    oldValues = uint16([0 0 0 0 0 0 0]);
end

history = uint16([0 0 0 0 0 0 0]);

for i=7:-1:2
    oldValues(i) = oldValues(i-1);
	history(i) = oldValues(i-1);
end
	
oldValues(1) = latest;
history(1) = latest;

== matlab function Trim Vals/Bufffer IC/Buffer IC Channel3 ==
  data: latest input inherited; history output inherited
function history = bufferICValues(latest)
% This block supports an embeddable subset of the MATLAB language.
% See the help menu for details. 

persistent oldValues;

if isempty(oldValues)
    oldValues = uint16([0 0 0 0 0 0 0]);
end

history = uint16([0 0 0 0 0 0 0]);

for i=7:-1:2
    oldValues(i) = oldValues(i-1);
	history(i) = oldValues(i-1);
end
	
oldValues(1) = latest;
history(1) = latest;

== matlab function Inner Loop/ Navigation/Lateral Channel/myMux Fun3 ==
  data: u1 input inherited; y output inherited; u2 input inherited; u3 input inherited
function y = myMux(u1, u2, u3)
% This block supports an embeddable subset of the MATLAB language.
% See the help menu for details. 

y = [u1(1); u2(1); u3(1)];

== matlab function get Nav Vars/myMux Fun1 ==
  data: u1 input inherited; y output inherited; u2 input inherited; u3 input inherited
function y = myMux3(u1, u2, u3)
% This block supports an embeddable subset of the MATLAB language.
% See the help menu for details. 

y = [u1(1); u2(1); u3(1)];

== matlab function get Nav Vars/myMux Fun2 ==
  data: u1 input inherited; y output inherited; u2 input inherited
function y = myMux3(u1, u2)
% This block supports an embeddable subset of the MATLAB language.
% See the help menu for details. 

y = [u1(1:3); u2(1:3)];

== matlab function get Nav Vars/Euler Angles to Direction Cosine Matrix1/Create Transformation Matrix/myMux Fun1 ==
  data: u1 input inherited; y output inherited; u2 input inherited; u3 input inherited; u4 input inherited; u5 input inherited; u6 input inherited; u7 input inherited; u8 input inherited; u9 input inherited
function y = myMux3(u1, u2, u3, u4, u5, u6, u7, u8, u9)
% This block supports an embeddable subset of the MATLAB language.
% See the help menu for details. 

y = [u1(1); u2(1); u3(1);u4(1); u5(1); u6(1); u7(1); u8(1); u9(1)];

== matlab function get Nav Vars/Euler Angles to Direction Cosine Matrix2/Create Transformation Matrix/myMux Fun1 ==
  data: u1 input inherited; y output inherited; u2 input inherited; u3 input inherited; u4 input inherited; u5 input inherited; u6 input inherited; u7 input inherited; u8 input inherited; u9 input inherited
function y = myMux3(u1, u2, u3, u4, u5, u6, u7, u8, u9)
% This block supports an embeddable subset of the MATLAB language.
% See the help menu for details. 

y = [u1(1); u2(1); u3(1);u4(1); u5(1); u6(1); u7(1); u8(1); u9(1)];

== matlab function get Nav Vars/Euler Angles to Direction Cosine Matrix1/Subsystem5/myMux Fun1 ==
  data: u1 input inherited; y output inherited; u2 input inherited; u3 input inherited
function y = myMux3(u1, u2, u3)
% This block supports an embeddable subset of the MATLAB language.
% See the help menu for details. 

y = [u1(1); u2(1); u3(1)];

== matlab function get Nav Vars/Euler Angles to Direction Cosine Matrix1/Subsystem5/myMux Fun2 ==
  data: u1 input inherited; y output inherited; u2 input inherited; u3 input inherited
function y = myMux3(u1, u2, u3)
% This block supports an embeddable subset of the MATLAB language.
% See the help menu for details. 

y = [u1(1); u2(1); u3(1)];

== matlab function get Nav Vars/Euler Angles to Direction Cosine Matrix2/Subsystem5/myMux Fun1 ==
  data: u1 input inherited; y output inherited; u2 input inherited; u3 input inherited
function y = myMux3(u1, u2, u3)
% This block supports an embeddable subset of the MATLAB language.
% See the help menu for details. 

y = [u1(1); u2(1); u3(1)];

== matlab function get Nav Vars/Euler Angles to Direction Cosine Matrix2/Subsystem5/myMux Fun2 ==
  data: u1 input inherited; y output inherited; u2 input inherited; u3 input inherited
function y = myMux3(u1, u2, u3)
% This block supports an embeddable subset of the MATLAB language.
% See the help menu for details. 

y = [u1(1); u2(1); u3(1)];

== matlab function Inner Loop/ Navigation/Navigation/Park, Deyst & How Lat Accel Cmd/GainSchedule L2 and Get Groundspeed/negprotect1 ==
  data: val input inherited; zpVal output inherited
function zpVal = negProt(val)
% This block supports an embeddable subset of the MATLAB language.
% See the help menu for details. 

if val >= single(0.001)
    zpVal = val;
else
    zpVal = single(0.001);
end

== matlab function Inner Loop/ Navigation/Lateral Channel/0.5 sec  tau/Embedded MATLAB Function ==
  data: u input inherited; y output inherited; T input inherited; f input inherited
function y = fcn(u,T,f)
% This block supports an embeddable subset of the MATLAB language.
% See the help menu for details. 

persistent a
persistent b
persistent y_km1
persistent u_km1
if isempty(a)
    %tf = [T*omega/(2+T*omega) T*omega/(2+T*omega)],[1 (T*omega-2)/(T*omega+2)]
    %tf = [a a],[1 -b]
    omega = 2*pi*f;
    a=T*omega/(2+T*omega);
    b=-(T*omega-2)/(T*omega+2);
    y_km1=u;
    u_km1=u;
end

y = a*(u+u_km1)+b*y_km1;
y_km1=y;
u_km1=u;

== matlab function Inner Loop/ Navigation/Navigation/Compute WP Index/Switch when in Line Segment/Compute Total Run/Compute Distance/Norm/Subsystem3/Embedded MATLAB Function ==
  data: x input inherited; y input inherited; xDoty output inherited
function xDoty = myDot(x,y)
% This block supports an embeddable subset of the MATLAB language.
% See the help menu for details. 

xDoty = x(1)*y(1) + x(2)*y(2) + x(3)*y(3);

== matlab function Inner Loop/ Navigation/Navigation/Compute WP Index/Switch when in Line Segment/Compute Projection/Subsystem3/Embedded MATLAB Function ==
  data: x input inherited; y input inherited; xDoty output inherited
function xDoty = myDot(x,y)
% This block supports an embeddable subset of the MATLAB language.
% See the help menu for details. 

xDoty = x(1)*y(1) + x(2)*y(2) + x(3)*y(3);

== matlab function Inner Loop/ Navigation/Navigation/myMux Fun1 ==
  data: u1 input inherited; y output inherited; u2 input inherited; u3 input inherited
function y = myMux(u1, u2, u3)
% This block supports an embeddable subset of the MATLAB language.
% See the help menu for details. 

y = [u1(1); u2(1); u3(1)];

== matlab function Inner Loop/ Navigation/Navigation/Compute Lateral Error/Subsystem3/Embedded MATLAB Function ==
  data: x input inherited; y input inherited; xDoty output inherited
function xDoty = myDot(x,y)
% This block supports an embeddable subset of the MATLAB language.
% See the help menu for details. 

xDoty = x(1)*y(1) + x(2)*y(2) + x(3)*y(3);

== matlab function Inner Loop/ Navigation/Longitudinal Channel/5 sec tau for high speeds/Embedded MATLAB Function ==
  data: u input inherited; y output inherited; T input inherited; f input inherited
function y = fcn(u,T,f)
% This block supports an embeddable subset of the MATLAB language.
% See the help menu for details. 

persistent a
persistent b
persistent y_km1
persistent u_km1
if isempty(a)
    %tf = [T*omega/(2+T*omega) T*omega/(2+T*omega)],[1 (T*omega-2)/(T*omega+2)]
    %tf = [a a],[1 -b]
    omega = 2*pi*f;
    a=T*omega/(2+T*omega);
    b=-(T*omega-2)/(T*omega+2);
    y_km1=u;
    u_km1=u;
end

y = a*(u+u_km1)+b*y_km1;
y_km1=y;
u_km1=u;

== matlab function Inner Loop/ Navigation/Longitudinal Channel/0.3 sec  tau for low speeds/Embedded MATLAB Function ==
  data: u input inherited; y output inherited; T input inherited; f input inherited
function y = fcn(u,T,f)
% This block supports an embeddable subset of the MATLAB language.
% See the help menu for details. 

persistent a
persistent b
persistent y_km1
persistent u_km1
if isempty(a)
    %tf = [T*omega/(2+T*omega) T*omega/(2+T*omega)],[1 (T*omega-2)/(T*omega+2)]
    %tf = [a a],[1 -b]
    omega = 2*pi*f;
    a=T*omega/(2+T*omega);
    b=-(T*omega-2)/(T*omega+2);
    y_km1=u;
    u_km1=u;
end

y = a*(u+u_km1)+b*y_km1;
y_km1=y;
u_km1=u;
